simulink model "Model_of_pendulum_dynamics_for_SI_with_dryfriction_clean_4"  (R2023b)
settings: Solver=FixedStepAuto  StartTime=0.0  StopTime=T  FixedStep=step_size  RelTol=1e-6  AbsTol=1e-6
values from neighbouring files (symbols this model uses):
  A_in2 = scales2(NN)    [synthetic_data.m]
  Dth0 = 0    [synthetic_data.m]
  g = 9.81    [butterfly_real_data.m]    (also in synthetic_data.m)
  Kf = 0.001    [synthetic_data.m]
  NNN = 1+(iter-1)    [synthetic_data.m]
  Om_in2 = input_freq2(NN)    [synthetic_data.m]
  p1 = params(1)    [butterfly_real_data.m]    (also in synthetic_data.m)
  p2 = params(2)    [butterfly_real_data.m]    (also in synthetic_data.m)
  p3 = params(3)    [butterfly_real_data.m]    (also in synthetic_data.m)
  th0 = 0.01    [synthetic_data.m]
libraries: simulink x2
settings Model: Creator=shiriaev  LastModifiedBy=Artem
settings SolverCC: AlgebraicLoopSolver=TrustRegion
settings DebuggingCC: UnconnectedInputMsg=warning  UnconnectedOutputMsg=warning  UnconnectedLineMsg=warning
settings ModelReferenceCC: EnableRefExpFcnMdlSchedulingChecks=on

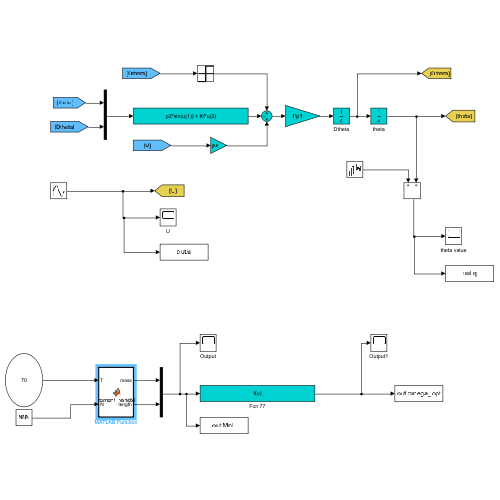
[thumbnail: Simulink's stored preview of the top-level diagram]
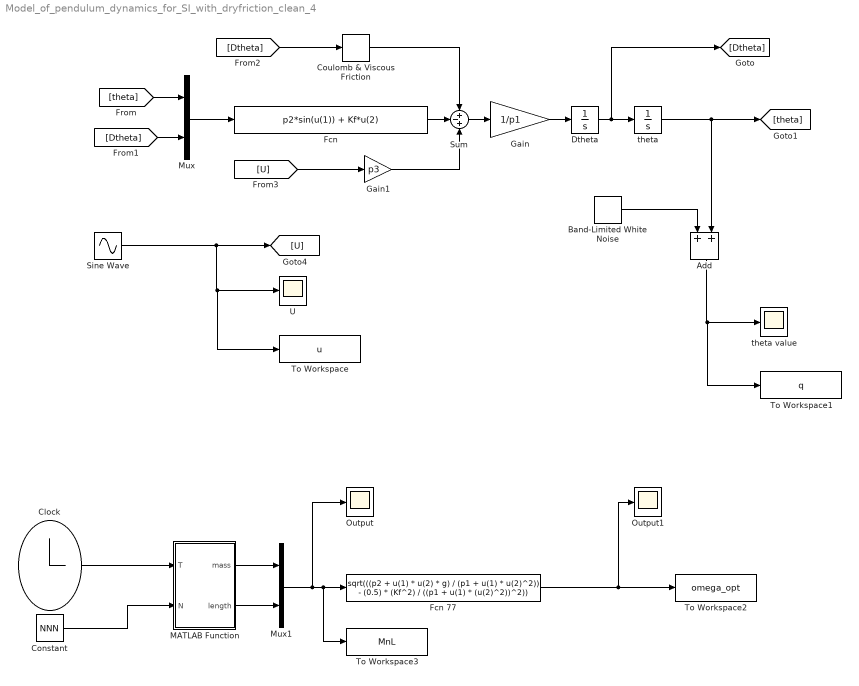
== system Model_of_pendulum_dynamics_for_SI_with_dryfriction_clean_4 ==
  Add : Sum
  Band-Limited White Noise : simulink/Sources/Band-Limited White Noise  Cov=[0.00000001]  Ts=0.01  seed=seed_rand
  Clock : Clock
      settings: Decimation=100
  Constant : Constant  Value=NNN
  Coulomb & Viscous Friction : simulink/Discontinuities/Coulomb & Viscous Friction  offset=0.00000005  gain=0
  Dtheta : Integrator  InitialCondition=Dth0
  Fcn : Fcn  Expr=p2*sin(u(1)) + Kf*u(2)
  Fcn 77 : Fcn  Expr=sqrt(((p2 + u(1) * u(2) * g) / (p1 + u(1) * u(2)^2)) - (0.5) * (Kf^2) / ((p1 + u(1) * (u(2)^2))^2))
  Gain : Gain  Gain=1/p1
  Gain1 : Gain  Gain=p3
  MATLAB Function : MATLAB Function  TreatAsAtomicUnit=on
  Mux : Mux  Inputs=2
  Mux1 : Mux  Inputs=2
  Output : Scope
  Output1 : Scope
  Sine Wave : Sin  Amplitude=A_in2  Frequency=Om_in2  SampleTime=0
  Sum : Sum  Inputs=+-+
  To Workspace : ToWorkspace  VariableName=u  SaveFormat=Timeseries  SampleTime=-1
  To Workspace1 : ToWorkspace  VariableName=q  SaveFormat=Timeseries  SampleTime=-1
  To Workspace2 : ToWorkspace  VariableName=omega_opt  SaveFormat=Timeseries  SampleTime=-1
  To Workspace3 : ToWorkspace  VariableName=MnL  SaveFormat=Timeseries  SampleTime=-1
  U : Scope
  theta : Integrator  InitialCondition=th0
  theta value : Scope
  wires:
  Dtheta/1 -> [Dtheta], theta/1
  theta/1 -> Add/2, [theta]
  [theta] -> Mux/1
  [Dtheta] -> Mux/2
  Mux/1 -> Fcn/1
  Gain/1 -> Dtheta/1
  Sum/1 -> Gain/1
  [U] -> Gain1/1
  Sine Wave/1 -> To Workspace/1, U/1, [U]
  [Dtheta] -> Coulomb & Viscous Friction/1
  Coulomb & Viscous Friction/1 -> Sum/1
  Fcn/1 -> Sum/2
  Gain1/1 -> Sum/3
  Band-Limited White Noise/1 -> Add/1
  Add/1 -> To Workspace1/1, theta value/1
  Fcn 77/1 -> Output1/1, To Workspace2/1
  Mux1/1 -> Output/1, To Workspace3/1, Fcn 77/1
  MATLAB Function/1(mass) -> Mux1/1
  MATLAB Function/2(length) -> Mux1/2
  Clock/1 -> MATLAB Function/1(T)
  Constant/1 -> MATLAB Function/2(N)

== matlab function Model_of_pendulum_dynamics_for_SI_with_dryfriction_clean_4/MATLAB Function ==
  settings: updateMethod=DISCRETE
  data: T input; mass output; length output; N input
% function [mass, length] = increment_variables(T)
%     % u is the simulation time input (from the Clock block or similar)
% 
%     % Persistent variables to store the current values of mass and length
%     persistent current_mass current_length
% 
%     % Initial conditions (starting values for mass and length)
%     if isempty(current_mass)
%         current_mass = 0.1;  % Initial mass
%     end
% 
%     if isempty(current_length)
%         current_length = 0.05;  % Initial length
%     end
% 
%     timez = 10;
%     % Define the step sizes for mass and length
%     mass_step_size = 0.1*timez;  % Change in mass per time step
%     length_step_size = 0.05*timez;  % Change in length per time step
% 
%     % Calculate the time intervals for updates
%     N = 3;
%     total_time = 70;
%     interval = total_time / N;
% 
%     % Update the mass and length at the end of each interval
%     if T >= interval && T < 2 * interval
%         current_mass = 1 * mass_step_size;
%         current_length = 1 * length_step_size;
%     elseif T >= 2 * interval && T < 3 * interval
%         current_mass = 2 * mass_step_size;
%         current_length = 2 * length_step_size;
%     elseif T >= 3 * interval
%         current_mass = 3 * mass_step_size;
%         current_length = 3 * length_step_size;
%     end
%     % Output the updated mass and length
%     mass = current_mass;
%     length = current_length;
% end



function [mass, length] = increment_variables(T,N)
    % Total time of the experiment
    %total_time = 70; 

    % Number of updates (e.g., 3 updates)
    N_1 = N;

    % Persistent variables to store the current values of mass and length
    persistent current_mass current_length

    % Initial conditions (starting values for mass and length)
    if isempty(current_mass)
        current_mass = 0;  % Initial mass
    end

    if isempty(current_length)
        current_length = 0;  % Initial length
    end

    % Define the step sizes for mass and length
    mass_step_size = 0.05;  % Total change in mass over T time
    length_step_size = 0.005;  % Total change in length over T time

    % Calculate the time intervals for updates
    %interval = total_time / N_1;
    
    % Determine which step we are currently in
    %step_number = min(floor(T / interval) + 1, N_1);
    
    % Update the mass and length based on the current step number
    %current_mass = step_number * mass_step_size;
    %current_length = step_number * length_step_size;

    % Output the updated mass and length
    mass = mass_step_size*(N_1-1) ;
    length =  length_step_size*(N_1-1) ;
end
